simulink model "PROJETOFINALmotor"  (R2021a)
settings: Solver=VariableStepAuto  StartTime=0  StopTime=144  FixedStep=0.1  RelTol=1e-3
model workspace (MAT data in the model file):
  variavelteste = 0
libraries: autolibsharedmappedengines x2, spsACVoltageSourceLib x1, spsCurrentMeasurementLib x1, spsSeriesRLCBranchLib x1, spspowerguiLib x1
(part 4 of 4)

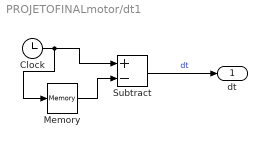
== system PROJETOFINALmotor/dt1 ==
  Clock : Clock
  Memory : Memory
  Subtract : Sum  Inputs=+-
  dt : Outport
  wires:
  Memory/1 -> Subtract/2
  Clock/1 -> Memory/1, Subtract/1
  Subtract/1 -> dt/1  "dt"

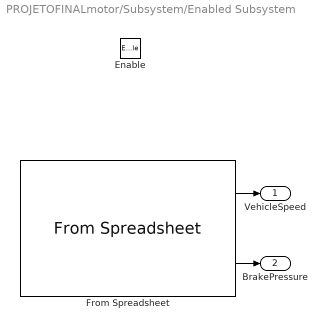
== system PROJETOFINALmotor/Subsystem/Enabled Subsystem ==
  Enable : EnablePort
  From Spreadsheet : FromSpreadsheet  FileName=C:\Users\Henrique\Downloads\tempo.xlsx  SheetName=tempo  Range=A1:C1441  SampleTime=-1
  VehicleSpeed : Outport  InitialOutput=0  VectorParamsAs1DForOutWhenUnconnected=off
  BrakePressure : Outport  Port=2  InitialOutput=0  VectorParamsAs1DForOutWhenUnconnected=off
  wires:
  From Spreadsheet/1 -> VehicleSpeed/1
  From Spreadsheet/2 -> BrakePressure/1

== matlab function PROJETOFINALmotor/Subsystem/Inverte Sinal do torque aceleraçãoXdesaceleração ==
  data: EngTrq input; EngTrqSaida output; derivada input
function EngTrqSaida = SinalDoTorque(EngTrq,derivada)

%derivada positiva sinal positivo, derivada negativa sinal de saida
%negativo

if (derivada>0)  
    EngTrqSaida = EngTrq;
else 
    EngTrqSaida = -EngTrq;
end

== matlab function PROJETOFINALmotor/Câmbio/MATLAB Function1 ==
  data: Marcha input; PosicaoMarcha output; Char output
function [PosicaoMarcha,Char] = ConverterMarcha(Marcha)

if Marcha == 'P'
    PosicaoMarcha = 1; 
    Char = uint8(80);
elseif Marcha == 'N'
    PosicaoMarcha = 2; 
    Char = uint8(78);
elseif Marcha == 'D'
    PosicaoMarcha = 3; 
    Char = uint8(68);
elseif Marcha == 'R'
    PosicaoMarcha = 4; 
    Char = uint8(82);
else 
    PosicaoMarcha = 0;
    Char = uint8(69);
end

== stateflow chart PROJETOFINALmotor/Sistema Ar Condicionado/Chart1 ==
  state AC_Normal
    entry:
    AC_OK = 1;
  state AC_Block
    entry:
    AC_OK = 0;
  (default) -> AC_Normal
  AC_Block -> AC_Normal : [abs(CabinTemperature - TargetTemperature) <= delta]
  AC_Normal -> AC_Block : [abs(CabinTemperature - TargetTemperature) > delta]
  data: CabinTemperature input; TargetTemperature input double; delta input; AC_OK output double

== matlab function PROJETOFINALmotor/Subsystem/MATLAB Function ==
  data: Marcha input; Ativar output; EngineSwitch input
function Ativar = AtivarSubSistema(Marcha,EngineSwitch)

%A marcha igual a 3 significa que o carro está no "D" - Modo Drive

if ((Marcha==3) && (EngineSwitch==1))  
    Ativar = 1;
else 
    Ativar = 0;
end

== stateflow chart PROJETOFINALmotor/Start Stop/Chart ==
  state EngineON1
    entry:
    EngineState = 1;  % Motor ligado
    tempo_minimo_ligado = 0;  % Reseta o contador ao entrar no estado
    during:
    tempo_minimo_ligado = tempo_minimo_ligado + dt;  % Incrementa usando dt real da simulação
  state EngineOFF1
    EngineState = 0;  % Motor desligado
  state AutoStop1
    EngineState = 0;  % Motor desligado temporariamente
  EngineON1 -> EngineOFF1 [order 1] : [EngineSwitch == 0
      | ]
  EngineOFF1 -> EngineON1 : [EngineSwitch == 1
      | ]
  AutoStop1 -> EngineON1 : [(BrakePressure < 0.2) || (AC_OK == 0) || (DoorStatus == 0) || (SeatBeltStatus == 0) || (BattVoltage < 12) || (EPBStatus == 1) || (GearPos == 1) || (GearPos == 4)
      | ]
  EngineON1 -> AutoStop1 [order 2] : [((GearPos == 3) || (GearPos == 2)) && (BrakePressure > 0.7) && (VehicleSpeed==0) && (EngineTemperature > 80) && (AC_OK == 1) && (BattVoltage > 12) && (DoorStatus == 1) && (EPBStatus == 0) && (SeatBeltStatus == 1) && (HoodStatus == 1) ]
  (default) -> EngineOFF1
  data: VehicleSpeed input; BrakePressure input; THRPEDAL input; SeatBeltStatus input; HoodStatus input; DoorStatus input; GearPos input; EPBStatus input; EngineState output double; EngineSwitch input double; tempo_minimo_ligado local double =0; dt input =0.01; BattVoltage input; EngineTemperature input; AC_OK input
